simulink model "APP_PlausBrk"  (R2016b)
settings: configuration reference "CodeGenConfigSet" (kept outside this file)
values from neighbouring files (symbols this model uses):
  APP_drUnFltLim_C = Calibration.Parameter    [init_APP_PlausBrk.m]
  APP_nLim_C = Calibration.Parameter    [init_APP_PlausBrk.m]
  APP_swtAppGradEna_C = Calibration.Parameter    [init_APP_PlausBrk.m]
  APP_swtBrkDet_C = Calibration.Parameter    [init_APP_PlausBrk.m]
  APP_swtRstCon_C = Calibration.Parameter    [init_APP_PlausBrk.m]
  APP_tiGradCondDebHiLo_C = Calibration.Parameter    [init_APP_PlausBrk.m]
  APP_tiGradCondDebLoHi_C = Calibration.Parameter    [init_APP_PlausBrk.m]
  APP_tiPlaBrkDetDeb_C = Calibration.Parameter    [init_APP_PlausBrk.m]
  APP_tiPlaBrkRstDeb_C = Calibration.Parameter    [init_APP_PlausBrk.m]
  APP_vLim_C = Calibration.Parameter    [init_APP_PlausBrk.m]
undefined symbols (not defined in the file or in its folder): AccPedal_switch_conv, APP_PlausBrk_DT, Switch_conv
libraries: CXLib x9
settings Model: Creator=lenovo  LastModifiedBy=lenovo
settings ConfigSetRef: SourceLocation=Base Workspace

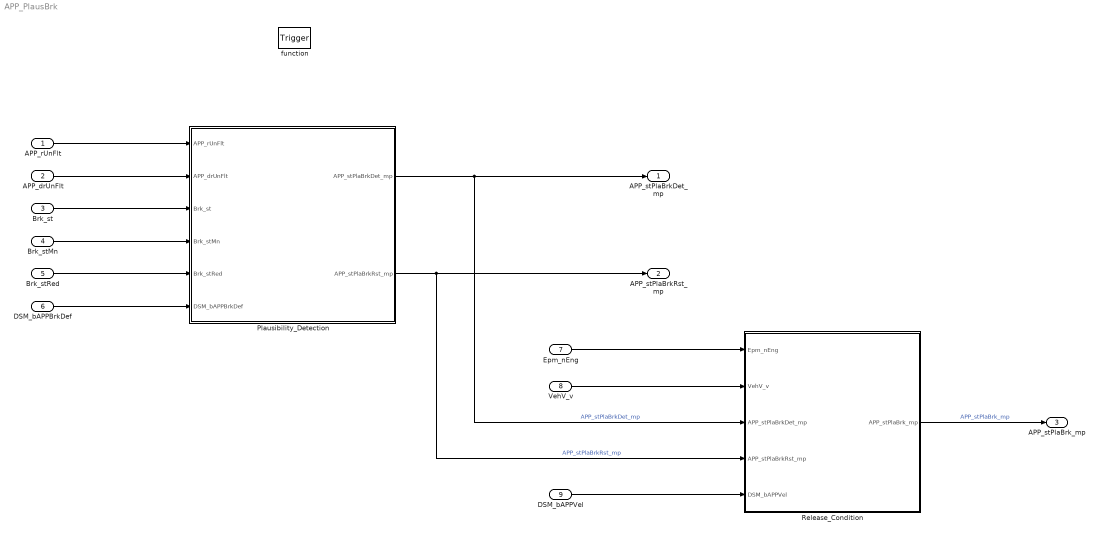
== system APP_PlausBrk ==
  APP_rUnFlt : Inport  Tag=%  Description=Unfiltered APP value  OutMin=0  OutMax=100  OutDataTypeStr=Accpedal_rate
  APP_drUnFlt : Inport  Tag=%/s  Description=Acceleration pedal position gradient of unfilterd value  Port=2  OutMin=-399  OutMax=399  OutDataTypeStr=Accpedal_rate_s
  Brk_st : Inport  Description=Brake switch state  Port=3  OutMin=0  OutMax=255  OutDataTypeStr=State_uint8
  Brk_stMn : Inport  Description=Status of the main brake  Port=4  OutMin=0  OutMax=1  OutDataTypeStr=boolean
  Brk_stRed : Inport  Description=Status of the redundant break  Port=5  OutMin=0  OutMax=1  OutDataTypeStr=boolean
  DSM_bAPPBrkDef : Inport  Description=status of FId_APPBrkDef  Port=6  OutMin=0  OutMax=1  OutDataTypeStr=boolean
  Epm_nEng : Inport  Tag=rpm  Description=Engine speed  Port=7  OutMin=0  OutMax=6000  OutDataTypeStr=EngSpeed_rpm
  VehV_v : Inport  Tag=km/h  Description=Vehicle speed  Port=8  OutMin=0  OutMax=250  OutDataTypeStr=VehSpeed_km_h
  DSM_bAPPVel : Inport  Description=status of FId_APPVel  Port=9  OutMin=0  OutMax=1  OutDataTypeStr=boolean
  function : TriggerPort  TriggerType=function-call  VariantControl=Variant
  Plausibility_Detection : Subsystem
  Release_Condition : Subsystem
  APP_stPlaBrkDet_mp : Outport  Description=State of detection plausibility with brake  OutMin=0  OutMax=1  OutDataTypeStr=boolean
  APP_stPlaBrkRst_mp : Outport  Description=State of reset plausibility with brake  Port=2  OutMin=0  OutMax=1  OutDataTypeStr=boolean
  APP_stPlaBrk_mp : Outport  Description=State of plausibility APP with brake  Port=3  OutMin=0  OutMax=1  OutDataTypeStr=boolean
  wires:
  Release_Condition/1(APP_stPlaBrk_mp) -> APP_stPlaBrk_mp/1  "APP_stPlaBrk_mp"
  VehV_v/1 -> Release_Condition/2(VehV_v)
  Epm_nEng/1 -> Release_Condition/1(Epm_nEng)
  DSM_bAPPVel/1 -> Release_Condition/5(DSM_bAPPVel)
  APP_rUnFlt/1 -> Plausibility_Detection/1(APP_rUnFlt)
  APP_drUnFlt/1 -> Plausibility_Detection/2(APP_drUnFlt)
  Brk_st/1 -> Plausibility_Detection/3(Brk_st)
  Brk_stMn/1 -> Plausibility_Detection/4(Brk_stMn)
  Brk_stRed/1 -> Plausibility_Detection/5(Brk_stRed)
  DSM_bAPPBrkDef/1 -> Plausibility_Detection/6(DSM_bAPPBrkDef)
  Plausibility_Detection/1(APP_stPlaBrkDet_mp) -> APP_stPlaBrkDet_mp/1, Release_Condition/3(APP_stPlaBrkDet_mp)  "APP_stPlaBrkDet_mp"
  Plausibility_Detection/2(APP_stPlaBrkRst_mp) -> APP_stPlaBrkRst_mp/1, Release_Condition/4(APP_stPlaBrkRst_mp)  "APP_stPlaBrkRst_mp"

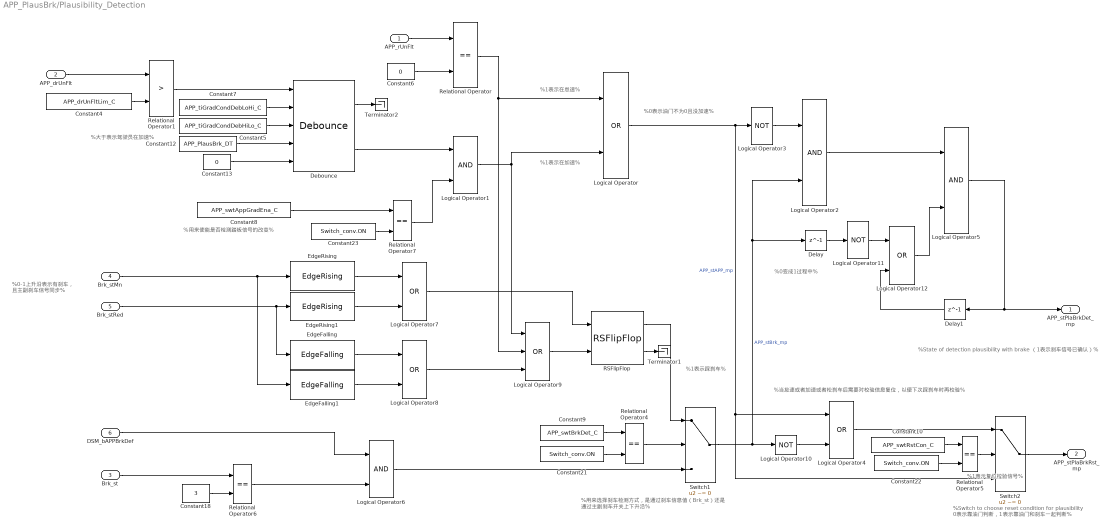
== system APP_PlausBrk/Plausibility_Detection ==
  note: %用来选择刹车检测方式，是通过刹车信息值（Brk_st）还是
      | 通过主副刹车开关上下升沿%
  note: %用来使能是否检测踏板信号的改变%
  note: %大于表示驾驶员在加速%
  note: %State of detection plausibility with brake（1表示刹车信号已确认）%
  note: %1表示复位校验信号%
  note: %Switch to choose reset condition for plausibility
      | 0表示靠油门判断，1表示靠油门和刹车一起判断%
  note: %0-1上升沿表示有刹车，
      | 且主副刹车信号同步%
  note: %1表示在加速%
  note: %1表示踩刹车%
  note: %当怠速或者加速或者松刹车后需要对校验信息复位，以便下次踩刹车时再校验%
  note: %0变成1过程中%
  note: %0表示油门不为0且没加速%
  note: %1表示在怠速%
  APP_rUnFlt : Inport  Tag=%  Description=Unfiltered APP value  OutMin=0  OutMax=100  OutDataTypeStr=Accpedal_rate
  APP_drUnFlt : Inport  Tag=%  Description=Acceleration pedal position gradient of unfilterd value  Port=2  OutMin=-200  OutMax=200  OutDataTypeStr=Accpedal_rate_s
  Brk_st : Inport  Tag=-  Description=Brake switch state  Port=3  OutMin=0  OutMax=255  OutDataTypeStr=State_uint8
  Brk_stMn : Inport  Tag=-  Description=Status of the main brake  Port=4  OutMin=0  OutMax=1  OutDataTypeStr=boolean
  Brk_stRed : Inport  Tag=-  Description=Status of the redundant break  Port=5  OutMin=0  OutMax=1  OutDataTypeStr=boolean
  DSM_bAPPBrkDef : Inport  Tag=-  Description=status of FId_APPBrkDef  Port=6  OutMin=0  OutMax=1  OutDataTypeStr=boolean
  Constant10 : Constant  RequirementInfo={'other' 'APP_requirements.doc' '@Simulink_requirement_item_17' 'true' '刹车校验结果复位。' '' ; 'other' 'APP_requirements.doc' '@Simulink_requirement_item_18' 'true' '刹车校验使能条件。' '' } %GIDa_7cdf6729_fcb9_4cb7_82d1_22154a608f76  Value=APP_swtRstCon_C
  Constant12 : Constant  Value=APP_PlausBrk_DT  OutDataTypeStr=Inherit: Inherit via back propagation
  Constant13 : Constant  Value=0  OutDataTypeStr=boolean
  Constant18 : Constant  Value=3  OutDataTypeStr=Inherit: Inherit via back propagation
  Constant21 : Constant  Value=Switch_conv.ON  OutDataTypeStr=Inherit: Inherit via back propagation
  Constant22 : Constant  Value=Switch_conv.ON  OutDataTypeStr=Inherit: Inherit via back propagation
  Constant23 : Constant  Value=Switch_conv.ON  OutDataTypeStr=Inherit: Inherit via back propagation
  Constant4 : Constant  RequirementInfo={'other' 'APP_requirements.doc' '@Simulink_requirement_item_14' 'true' '油门加速检测。' '' } %GIDa_ada3c8d9_0be7_4473_bf6b_866c273a3fa6  Value=APP_drUnFltLim_C
  Constant5 : Constant  Value=APP_tiGradCondDebHiLo_C
  Constant6 : Constant  Value=0  OutDataTypeStr=Inherit: Inherit via back propagation
  Constant7 : Constant  Value=APP_tiGradCondDebLoHi_C
  Constant8 : Constant  Value=APP_swtAppGradEna_C
  Constant9 : Constant  Value=APP_swtBrkDet_C
  Debounce : CXLib/Debounce  RequirementInfo={'other' 'APP_requirements.doc' '@Simulink_requirement_item_14' 'true' '油门加速检测。' '' } %GIDa_b4698ea0_19ba_45c5_9428_195d88eeda08
  Delay : Delay  RequirementInfo={'other' 'APP_requirements.doc' '@Simulink_requirement_item_16' 'true' '刹车校验结果确认。' '' } %GIDa_5923b175_2d2c_4a14_93ad_71d2e05f14da  DelayLength=1  InitialCondition=0
  Delay1 : Delay  RequirementInfo={'other' 'APP_requirements.doc' '@Simulink_requirement_item_16' 'true' '刹车校验结果确认。' '' } %GIDa_d7afd61e_c143_4619_b2ca_83431966e189  DelayLength=1  InitialCondition=0
  EdgeFalling : CXLib/EdgeFalling  RequirementInfo={'other' 'APP_requirements.doc' '@Simulink_requirement_item_15' 'true' '主副刹车信号校验。' '' ; 'other' 'APP_requirements.doc' '@Simulink_requirement_item_16' 'true' '刹车校验结果确认。' '' } %GIDa_9c9e410b_9812_487f_8607_3ceb6f43c261
  EdgeFalling1 : CXLib/EdgeFalling  RequirementInfo={'other' 'APP_requirements.doc' '@Simulink_requirement_item_15' 'true' '主副刹车信号校验。' '' ; 'other' 'APP_requirements.doc' '@Simulink_requirement_item_16' 'true' '刹车校验结果确认。' '' } %GIDa_8a2f73da_f6e8_4145_98ff_4125aed9f786
  EdgeRising : CXLib/EdgeRising  RequirementInfo={'other' 'APP_requirements.doc' '@Simulink_requirement_item_15' 'true' '主副刹车信号校验。' '' ; 'other' 'APP_requirements.doc' '@Simulink_requirement_item_16' 'true' '刹车校验结果确认。' '' } %GIDa_130cd836_14c9_4d65_b578_8bf021f58f29
  EdgeRising1 : CXLib/EdgeRising  RequirementInfo={'other' 'APP_requirements.doc' '@Simulink_requirement_item_15' 'true' '主副刹车信号校验。' '' ; 'other' 'APP_requirements.doc' '@Simulink_requirement_item_16' 'true' '刹车校验结果确认。' '' } %GIDa_7e719b6f_07df_4367_8793_80782af06983
  Logical Operator : Logic  Operator=OR  OutDataTypeStr=boolean
  Logical Operator1 : Logic  OutDataTypeStr=boolean
  Logical Operator10 : Logic  Operator=NOT  AllPortsSameDT=off  OutDataTypeStr=boolean
  Logical Operator11 : Logic  RequirementInfo={'other' 'APP_requirements.doc' '@Simulink_requirement_item_16' 'true' '刹车校验结果确认。' '' } %GIDa_6dd49488_3038_4eee_b376_a204f75dcde4  Operator=NOT  AllPortsSameDT=off  OutDataTypeStr=boolean
  Logical Operator12 : Logic  RequirementInfo={'other' 'APP_requirements.doc' '@Simulink_requirement_item_16' 'true' '刹车校验结果确认。' '' } %GIDa_7a714cd9_d80c_4a73_8bc7_29757852b14a  Operator=OR  OutDataTypeStr=boolean
  Logical Operator2 : Logic  RequirementInfo={'other' 'APP_requirements.doc' '@Simulink_requirement_item_16' 'true' '刹车校验结果确认。' '' } %GIDa_87b31cb2_dc57_4b30_9afb_17704f44ae05  OutDataTypeStr=boolean
  Logical Operator3 : Logic  Operator=NOT  AllPortsSameDT=off  OutDataTypeStr=boolean
  Logical Operator4 : Logic  RequirementInfo={'other' 'APP_requirements.doc' '@Simulink_requirement_item_17' 'true' '刹车校验结果复位。' '' ; 'other' 'APP_requirements.doc' '@Simulink_requirement_item_18' 'true' '刹车校验使能条件。' '' } %GIDa_7f7a4271_120f_4da7_b1c2_4f0564aa2087  Operator=OR  OutDataTypeStr=boolean
  Logical Operator5 : Logic  RequirementInfo={'other' 'APP_requirements.doc' '@Simulink_requirement_item_16' 'true' '刹车校验结果确认。' '' } %GIDa_ca627c2c_c3b8_421d_9b42_25a9bfef9d31  OutDataTypeStr=boolean
  Logical Operator6 : Logic  OutDataTypeStr=boolean
  Logical Operator7 : Logic  RequirementInfo={'other' 'APP_requirements.doc' '@Simulink_requirement_item_15' 'true' '主副刹车信号校验。' '' ; 'other' 'APP_requirements.doc' '@Simulink_requirement_item_16' 'true' '刹车校验结果确认。' '' } %GIDa_cafec61c_4236_456d_b17a_3fa3ad24098d  Operator=OR  OutDataTypeStr=boolean
  Logical Operator8 : Logic  RequirementInfo={'other' 'APP_requirements.doc' '@Simulink_requirement_item_15' 'true' '主副刹车信号校验。' '' ; 'other' 'APP_requirements.doc' '@Simulink_requirement_item_16' 'true' '刹车校验结果确认。' '' } %GIDa_fe08a414_27fb_4f91_9582_d25debc7b1c1  Operator=OR  OutDataTypeStr=boolean
  Logical Operator9 : Logic  RequirementInfo={'other' 'APP_requirements.doc' '@Simulink_requirement_item_15' 'true' '主副刹车信号校验。' '' ; 'other' 'APP_requirements.doc' '@Simulink_requirement_item_16' 'true' '刹车校验结果确认。' '' } %GIDa_3fa06d14_e2d0_4725_8a21_7fe9df434943  Operator=OR  Inputs=3  OutDataTypeStr=boolean
  RSFlipFlop : CXLib/RSFlipFlop  RequirementInfo={'other' 'APP_requirements.doc' '@Simulink_requirement_item_15' 'true' '主副刹车信号校验。' '' ; 'other' 'APP_requirements.doc' '@Simulink_requirement_item_16' 'true' '刹车校验结果确认。' '' } %GIDa_50ce1de4_26c0_42a5_a9fe_e26c49cb565f
  Relational Operator{,4..7} (5 alike) : RelationalOperator  Operator===  OutDataTypeStr=boolean  RndMeth=Nearest  InputSameDT=on
  Relational Operator1 : RelationalOperator  RequirementInfo={'other' 'APP_requirements.doc' '@Simulink_requirement_item_14' 'true' '油门加速检测。' '' } %GIDa_126c7342_844e_4705_896e_33ea271e9e62  Operator=>  OutDataTypeStr=boolean  RndMeth=Nearest  InputSameDT=on
  Switch1 : Switch  Criteria=u2 ~= 0  Threshold=AccPedal_switch_conv.OFF  InputSameDT=on
  Switch2 : Switch  RequirementInfo={'other' 'APP_requirements.doc' '@Simulink_requirement_item_17' 'true' '刹车校验结果复位。' '' ; 'other' 'APP_requirements.doc' '@Simulink_requirement_item_18' 'true' '刹车校验使能条件。' '' } %GIDa_5dab3ebf_fb30_474e_888e_6b0f8d38a92c  Criteria=u2 ~= 0  InputSameDT=on
  Terminator1 : Terminator
  Terminator2 : Terminator
  APP_stPlaBrkDet_mp : Outport  Tag=-  Description=State of detection plausibility with brake  OutMin=0  OutMax=1  OutDataTypeStr=boolean
  APP_stPlaBrkRst_mp : Outport  Tag=-  Description=State of reset plausibility with brake  Port=2  OutMin=0  OutMax=1  OutDataTypeStr=boolean
  wires:
  Constant23/1 -> Relational Operator7/2
  Constant22/1 -> Relational Operator5/2
  Constant21/1 -> Relational Operator4/2
  Relational Operator4/1 -> Switch1/2
  DSM_bAPPBrkDef/1 -> Logical Operator6/1
  Brk_st/1 -> Relational Operator6/1
  Constant18/1 -> Relational Operator6/2
  Debounce/2 -> Logical Operator1/1
  Constant13/1 -> Debounce/5
  Constant12/1 -> Debounce/4
  Debounce/1 -> Terminator2/1
  Switch2/1 -> APP_stPlaBrkRst_mp/1
  Logical Operator5/1 -> APP_stPlaBrkDet_mp/1, Delay1/1
  Relational Operator6/1 -> Logical Operator6/2
  Relational Operator5/1 -> Switch2/2
  Relational Operator7/1 -> Logical Operator1/2
  RSFlipFlop/2 -> Terminator1/1
  Constant10/1 -> Relational Operator5/1
  Logical Operator4/1 -> Switch2/1
  Logical Operator10/1 -> Logical Operator4/2
  Logical Operator12/1 -> Logical Operator5/2
  Delay1/1 -> Logical Operator12/2
  Logical Operator11/1 -> Logical Operator12/1
  Delay/1 -> Logical Operator11/1
  Logical Operator2/1 -> Logical Operator5/1
  Switch1/1 -> Logical Operator10/1, Logical Operator2/2, Delay/1  "APP_stBrk_mp"
  Logical Operator6/1 -> Switch1/3
  RSFlipFlop/1 -> Switch1/1
  Logical Operator9/1 -> RSFlipFlop/2
  Logical Operator7/1 -> RSFlipFlop/1
  Logical Operator8/1 -> Logical Operator9/3
  EdgeFalling1/1 -> Logical Operator8/2
  EdgeFalling/1 -> Logical Operator8/1
  EdgeRising1/1 -> Logical Operator7/2
  EdgeRising/1 -> Logical Operator7/1
  Brk_stRed/1 -> EdgeRising1/1, EdgeFalling/1
  Brk_stMn/1 -> EdgeRising/1, EdgeFalling1/1
  Constant9/1 -> Relational Operator4/1
  Logical Operator3/1 -> Logical Operator2/1
  Logical Operator/1 -> Logical Operator3/1, Switch2/3, Logical Operator4/1  "APP_stAPP_mp"
  Logical Operator1/1 -> Logical Operator/2, Logical Operator9/1
  Constant8/1 -> Relational Operator7/1
  Constant5/1 -> Debounce/3
  Constant7/1 -> Debounce/2
  Relational Operator1/1 -> Debounce/1
  Constant6/1 -> Relational Operator/2
  Relational Operator/1 -> Logical Operator9/2, Logical Operator/1
  Constant4/1 -> Relational Operator1/2
  APP_drUnFlt/1 -> Relational Operator1/1
  APP_rUnFlt/1 -> Relational Operator/1

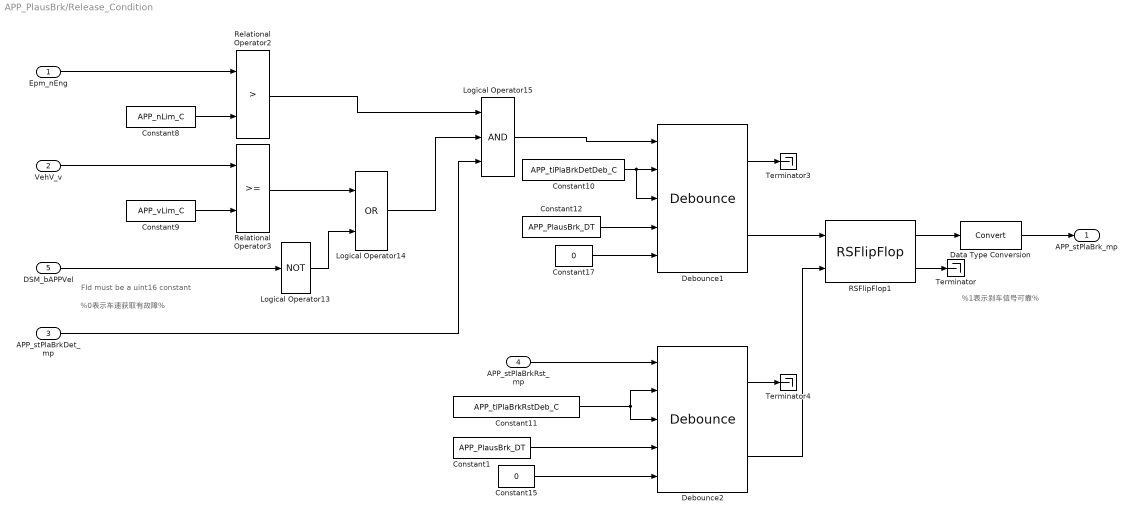
== system APP_PlausBrk/Release_Condition ==
  note: FId must be a uint16 constant
  note: %1表示刹车信号可靠%
  note: %0表示车速获取有故障%
  Epm_nEng : Inport  RequirementInfo={'other' 'APP_requirements.doc' '@Simulink_requirement_item_18' 'true' '刹车校验使能条件。' '' } %GIDa_ce191a20_4335_4d0e_b83c_894ec9b8de27
  VehV_v : Inport  RequirementInfo={'other' 'APP_requirements.doc' '@Simulink_requirement_item_18' 'true' '刹车校验使能条件。' '' } %GIDa_e430f071_ac83_4d87_a0d2_76173ba5b890  Port=2
  APP_stPlaBrkDet_mp : Inport  RequirementInfo={'other' 'APP_requirements.doc' '@Simulink_requirement_item_18' 'true' '刹车校验使能条件。' '' } %GIDa_0d65cc08_e528_4341_876c_b573ee694dde  Port=3
  APP_stPlaBrkRst_mp : Inport  RequirementInfo={'other' 'APP_requirements.doc' '@Simulink_requirement_item_18' 'true' '刹车校验使能条件。' '' } %GIDa_eb835b72_c785_4926_8375_d9a5112f57e1  Port=4
  DSM_bAPPVel : Inport  Tag=-  Description=status of FId_APPVel  Port=5  OutMin=0  OutMax=1
  Constant1 : Constant  Value=APP_PlausBrk_DT  OutDataTypeStr=Inherit: Inherit via back propagation
  Constant10 : Constant  Value=APP_tiPlaBrkDetDeb_C
  Constant11 : Constant  Value=APP_tiPlaBrkRstDeb_C
  Constant12 : Constant  Value=APP_PlausBrk_DT  OutDataTypeStr=Inherit: Inherit via back propagation
  Constant15 : Constant  Value=0  OutDataTypeStr=boolean
  Constant17 : Constant  Value=0  OutDataTypeStr=boolean
  Constant8 : Constant  RequirementInfo={'other' 'APP_requirements.doc' '@Simulink_requirement_item_18' 'true' '刹车校验使能条件。' '' } %GIDa_06615088_27b2_4a2b_8fff_531ba44218ea  Value=APP_nLim_C
  Constant9 : Constant  RequirementInfo={'other' 'APP_requirements.doc' '@Simulink_requirement_item_18' 'true' '刹车校验使能条件。' '' } %GIDa_ed84d778_cf65_4da2_973b_d3a63e525e63  Value=APP_vLim_C
  Data Type Conversion : DataTypeConversion
  Debounce1 : CXLib/Debounce  RequirementInfo={'other' 'APP_requirements.doc' '@Simulink_requirement_item_18' 'true' '刹车校验使能条件。' '' } %GIDa_b2158508_3669_4b5a_a44f_72e92b93bfae
  Debounce2 : CXLib/Debounce  RequirementInfo={'other' 'APP_requirements.doc' '@Simulink_requirement_item_17' 'true' '刹车校验结果复位。' '' ; 'other' 'APP_requirements.doc' '@Simulink_requirement_item_18' 'true' '刹车校验使能条件。' '' } %GIDa_b68598b8_2e9a_4630_8ab0_46ad845c33bd
  Logical Operator13 : Logic  Operator=NOT  AllPortsSameDT=off  OutDataTypeStr=boolean
  Logical Operator14 : Logic  RequirementInfo={'other' 'APP_requirements.doc' '@Simulink_requirement_item_18' 'true' '刹车校验使能条件。' '' } %GIDa_9538608e_4c90_4fd3_b83d_0011e7810137  Operator=OR  OutDataTypeStr=boolean
  Logical Operator15 : Logic  RequirementInfo={'other' 'APP_requirements.doc' '@Simulink_requirement_item_18' 'true' '刹车校验使能条件。' '' } %GIDa_54d9eef3_754f_4da6_8ef1_c57b9e7a8889  Inputs=3  OutDataTypeStr=boolean
  RSFlipFlop1 : CXLib/RSFlipFlop
  Relational Operator2 : RelationalOperator  RequirementInfo={'other' 'APP_requirements.doc' '@Simulink_requirement_item_18' 'true' '刹车校验使能条件。' '' } %GIDa_a4007579_2eed_4ced_8ea0_efa37f117194  Operator=>  OutDataTypeStr=boolean  RndMeth=Nearest  InputSameDT=on
  Relational Operator3 : RelationalOperator  RequirementInfo={'other' 'APP_requirements.doc' '@Simulink_requirement_item_18' 'true' '刹车校验使能条件。' '' } %GIDa_70f0f8cf_d829_4981_a407_8edcbbb0b650  OutDataTypeStr=boolean  RndMeth=Nearest  InputSameDT=on
  Terminator : Terminator
  Terminator3 : Terminator
  Terminator4 : Terminator
  APP_stPlaBrk_mp : Outport
  wires:
  APP_stPlaBrkRst_mp/1 -> Debounce2/1
  APP_stPlaBrkDet_mp/1 -> Logical Operator15/3
  Logical Operator13/1 -> Logical Operator14/2
  Data Type Conversion/1 -> APP_stPlaBrk_mp/1
  RSFlipFlop1/1 -> Data Type Conversion/1
  DSM_bAPPVel/1 -> Logical Operator13/1
  Debounce2/1 -> Terminator4/1
  Constant17/1 -> Debounce1/5
  Constant12/1 -> Debounce1/4
  Debounce1/1 -> Terminator3/1
  Constant15/1 -> Debounce2/5
  Constant1/1 -> Debounce2/4
  Constant8/1 -> Relational Operator2/2
  Constant9/1 -> Relational Operator3/2
  RSFlipFlop1/2 -> Terminator/1
  Debounce2/2 -> RSFlipFlop1/2
  Constant11/1 -> Debounce2/2, Debounce2/3
  Debounce1/2 -> RSFlipFlop1/1
  Constant10/1 -> Debounce1/2, Debounce1/3
  Logical Operator15/1 -> Debounce1/1
  Logical Operator14/1 -> Logical Operator15/2
  Relational Operator2/1 -> Logical Operator15/1
  Relational Operator3/1 -> Logical Operator14/1
  VehV_v/1 -> Relational Operator3/1
  Epm_nEng/1 -> Relational Operator2/1
